simulink model "task_2d"  (R2016a)
settings: Solver=VariableStepAuto  StartTime=0.0  StopTime=10.0  RelTol=1e-3
values from neighbouring files (symbols this model uses):
  a_phi1 = 3.6784    [model.mat]    (also in run_task_2d.m)
  a_phi2 = -0.7333    [model.mat]    (also in run_task_2d.m)
  g = 9.81    [model.mat]    (also in run_task_2d.m)
  Kd_phi = 3.03933954512    [model.mat]    (also in run_task_2d.m = (2*eta_phi*w_n_phi - a_phi1)/a_phi2)
  Ki_chi = 0.202820307377    [model.mat]    (also in run_task_2d.m = Wn_chi*Wn_chi*Vg/g)
  Ki_phi = -0.01    [model.mat]    (also in run_task_2d.m)
  Kp_chi = 4.27317564813    [model.mat]    (also in run_task_2d.m = 2*zeta_chi*Wn_chi*Vg/g)
  Kp_phi = -1.43333333333    [model.mat]    (also in run_task_2d.m = (delta_max_a*sign(a_phi2))/e_max_phi)
  Vg = 153.333333333    [model.mat]    (also in run_task_2d.m)
undefined symbols (not defined in the file or in its folder): sigbuilder_block
settings Model: Creator=marineac  LastModifiedBy=marineac

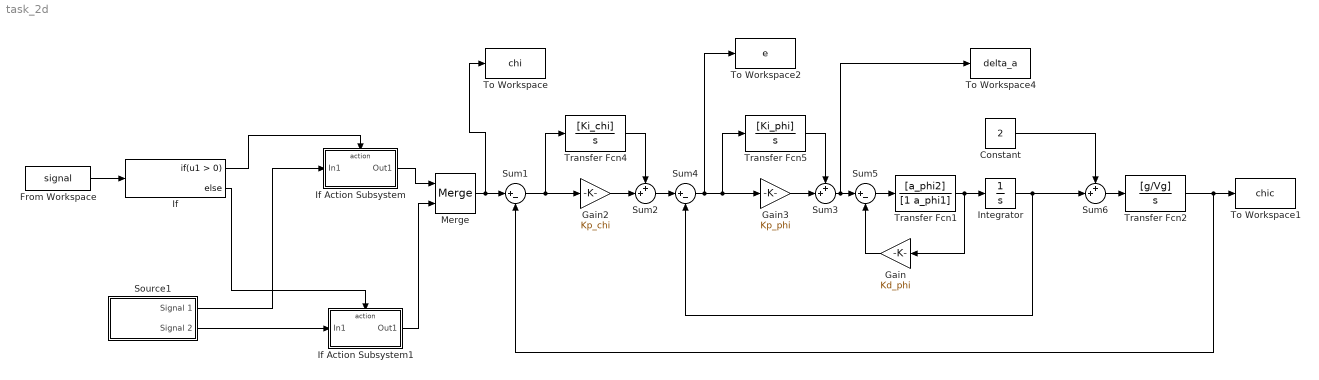
== system task_2d ==
  Constant : Constant  Value=2
  From Workspace : FromWorkspace  VariableName=signal  SampleTime=0
  Gain : Gain  Gain=Kd_phi
  Gain2 : Gain  Gain=Kp_chi
  Gain3 : Gain  Gain=Kp_phi
  If : If
  If Action Subsystem : Subsystem  TreatAsAtomicUnit=on
  If Action Subsystem1 : Subsystem  TreatAsAtomicUnit=on
  Integrator : Integrator
  Merge : Merge
  Source1 : Subsystem  Tag=STV Subsys  LoadFcn=sigbuilder_block('load');  StartFcn=sigbuilder_block('start');  StopFcn=sigbuilder_block('stop');  ClipboardFcn=sigbuilder_block('clipboard');  mask(Sigbuilder block){}
      mask help: Simulink:masks:SigbuilderBlock_MD
      mask init:
      | if ~strcmp(get_param(bdroot(gcbh),'SimulationStatus'),'stopped') tuvar = sigbuilder_block('maskInit'); end
      settings: CopyFcn=sigbuilder_block('copy');  DeleteFcn=sigbuilder_block('delete');  ModelCloseFcn=sigbuilder_block('modelClose');  PreSaveFcn=sigbuilder_block('preSave');  PauseFcn=sigbuilder_block('pause');  ContinueFcn=sigbuilder_block('continue');  NameChangeFcn=sigbuilder_block('namechange');  OpenFcn=sigbuilder_block('open',[45.75 30.75 891 673.5 ]);  CloseFcn=sigbuilder_block('close');
      mask Display: plot(0, 0, 100, 100,[2, 2, 32, 32, 2], [68, 8, 8, 68, 68],[32, 2], [38, 38], [32, 19, 2],[53, 60, 44], [32, 17, 17, 2],[16, 16, 31, 31]);txt = getActiveGroup(gcbh);text(2, 100, txt,'verticalAlignment', 'top');
  Sum1 : Sum  Inputs=|+-
  Sum2 : Sum  Inputs=++|
  Sum3 : Sum  Inputs=++|
  Sum4 : Sum  Inputs=|+-
  Sum5 : Sum  Inputs=|+-
  Sum6 : Sum  Inputs=++|
  To Workspace : ToWorkspace  VariableName=chi  SaveFormat=Timeseries  SampleTime=-1
  To Workspace1 : ToWorkspace  VariableName=chic  SaveFormat=Timeseries  SampleTime=-1
  To Workspace2 : ToWorkspace  VariableName=e  SaveFormat=Timeseries  SampleTime=-1
  To Workspace4 : ToWorkspace  VariableName=delta_a  SaveFormat=Timeseries  SampleTime=-1
  Transfer Fcn1 : TransferFcn  Numerator=[a_phi2]  Denominator=[1 a_phi1]
  Transfer Fcn2 : TransferFcn  Numerator=[g/Vg]  Denominator=[1 0]
  Transfer Fcn4 : TransferFcn  Numerator=[Ki_chi]  Denominator=[1 0]
  Transfer Fcn5 : TransferFcn  Numerator=[Ki_phi]  Denominator=[1 0]
  wires:
  Sum1/1 -> Gain2/1, Transfer Fcn4/1
  Transfer Fcn4/1 -> Sum2/1
  Gain2/1 -> Sum2/2
  Transfer Fcn5/1 -> Sum3/1
  Gain3/1 -> Sum3/2
  Sum2/1 -> Sum4/1
  Sum4/1 -> To Workspace2/1, Transfer Fcn5/1, Gain3/1
  Sum3/1 -> To Workspace4/1, Sum5/1
  Transfer Fcn1/1 -> Gain/1, Integrator/1
  Gain/1 -> Sum5/2
  Transfer Fcn2/1 -> To Workspace1/1, Sum1/2
  If Action Subsystem1/1(Out1) -> Merge/2
  Merge/1 -> To Workspace/1, Sum1/1
  If Action Subsystem/1(Out1) -> Merge/1
  Source1/2(Signal 2) -> If Action Subsystem1/1(In1)
  Source1/1(Signal 1) -> If Action Subsystem/1(In1)
  If/2 -> If Action Subsystem1/Action
  From Workspace/1 -> If/1
  If/1 -> If Action Subsystem/Action
  Sum5/1 -> Transfer Fcn1/1
  Integrator/1 -> Sum6/2, Sum4/2
  Constant/1 -> Sum6/1
  Sum6/1 -> Transfer Fcn2/1

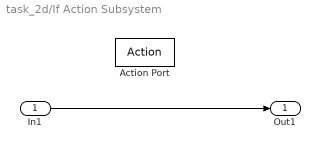
== system task_2d/If Action Subsystem ==
  In1 : Inport
  Action Port : ActionPort  ActionType=then
  Out1 : Outport
  wires:
  In1/1 -> Out1/1

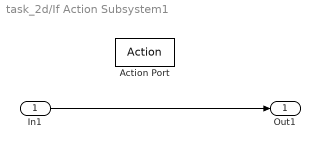
== system task_2d/If Action Subsystem1 ==
  In1 : Inport
  Action Port : ActionPort  ActionType=else
  Out1 : Outport
  wires:
  In1/1 -> Out1/1

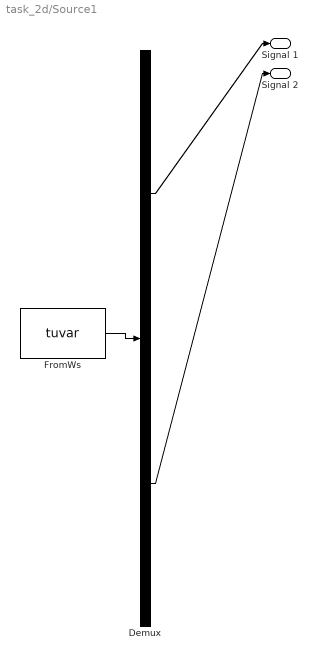
== system task_2d/Source1 ==
  Demux : Demux  Tag=STV Demux  Outputs=2
  FromWs : FromWorkspace  Tag=STV FromWs  VariableName=tuvar  SampleTime=0
      SigBuilderData=|
      | common.afterFinalStr = 'Extrapolate'
      | common.sampleTime = 0
      | dataSet.timeRange = [0 1000]
      | dataSet.name = 'Group 1'
      | sbobj.Groups.Name = 'Group 1'
      | sbobj.Groups.Signals(1).Name = 'Signal 1'
      | sbobj.Groups.Signals(1).XData = [0 201 201 386 386 550 550 700 700 1000]
      | sbobj.Groups.Signals(1).YData = [0 0 2.1 2.1 6.1 6.1 9.9 9.9 15.2 15.2]
      | sbobj.Groups.Signals(2).Name = 'Signal 2'
      | sbobj.Groups.Signals(2).XData = [0 76 86 92 100 116 122 128 136 144 156 226 232 236 242 254 260 262 268 300 414 422 428 434 440 442 450 464 472 478 486 494 500 512 528 661 671 678 684 691 698 704 794 800 806 810 814 826 1000]
      | sbobj.Groups.Signals(2).YData = [0 0 0.6 1.6 3 4.6 4.8 5 5 5 5 4.8 5.2 6.4 8.8 12.2 13.4 13.8 14.6 15.2 14.8 14.8 14.6 14.4 14 13.8 11.4 0.4 -0.2 -0.2 -0.2 -0.2 -0.2 -0.2 -0.4 -1.2 -1.6 -3 -8.4 -10 -10 -10 -10.2 -11.2 -13.6 -14.5 -14.8 -15 -14.5]
      | sbobj.Groups.TimeRange = [0 1000]
  Signal 1 : Outport  Tag=STV Outport
  Signal 2 : Outport  Tag=STV Outport  Port=2
  wires:
  FromWs/1 -> Demux/1
  Demux/1 -> Signal 1/1
  Demux/2 -> Signal 2/1
